simulink model "otomobil"  (Simulink 7.6)
settings: Solver=ode45  StartTime=0.0  StopTime=50  RelTol=1e-3
values from neighbouring files (symbols this model uses):
  co1 = 2500    [car.m]    (also in car_sis.m)
  co3 = 2500    [car.m]    (also in car_sis.m)
  co5 = 2500    [car.m]    (also in car_sis.m)
  co7 = 2500    [car.m]    (also in car_sis.m)
  dy = 0.007    [car.m]
  ko1 = 15000    [car.m]    (also in car_sis.m)
  ko2 = 250000    [car.m]    (also in car_sis.m)
  ko3 = 17000    [car.m]    (also in car_sis.m)
  ko4 = 250000    [car.m]    (also in car_sis.m)
  ko5 = 15000    [car.m]    (also in car_sis.m)
  ko6 = 250000    [car.m]    (also in car_sis.m)
  ko7 = 17000    [car.m]    (also in car_sis.m)
  ko8 = 250000    [car.m]    (also in car_sis.m)
  lo1 = 1.2    [car.m]
  lo2 = 1.4    [car.m]
  lo3 = 0.5    [car.m]
  lo4 = 1    [car.m]
  mo1 = 1100+80*4    (= 1420)    [car.m]    (also in car_sis.m = 1100)
  mo2 = 25    [car.m]    (also in car_sis.m)
  mo3 = 25    [car.m]    (also in car_sis.m = 45)
  mo4 = 45    [car.m]    (also in car_sis.m = 25)
  mo5 = 45    [car.m]    (also in car_sis.m)
  Vo = 50    [car.m]    (also in car_sis.m = 16.6666666667)
  wo = Vo/dy    (= 7142.85714286)    [car.m]
settings Model: Creator=user  LastModifiedBy=user

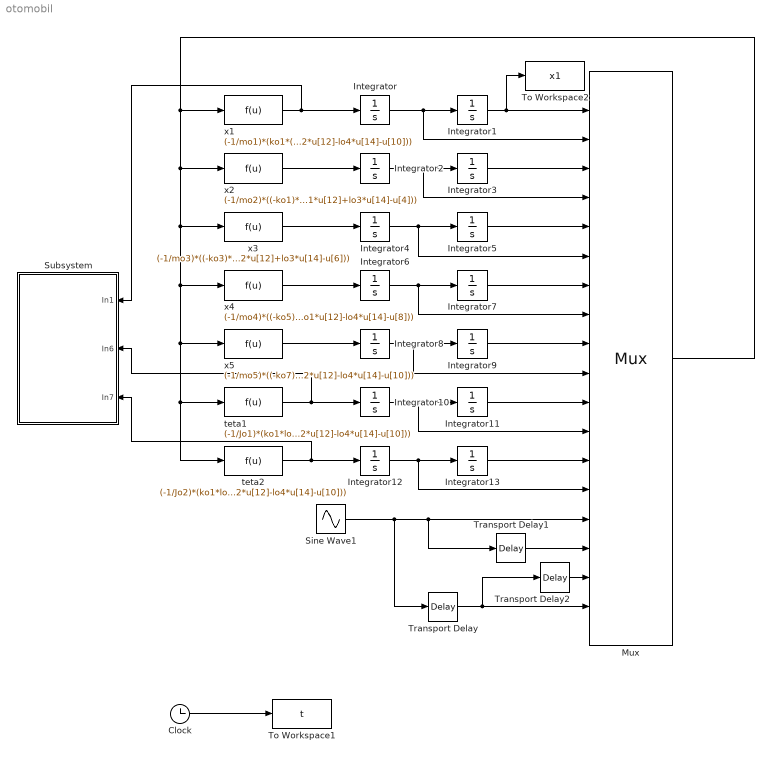
== system otomobil ==
  Clock : Clock
      settings: Decimation=10
  Integrator{,1..13} (14 alike) : Integrator
  Mux : Mux  Inputs=18
  Sine Wave1 : Sin  Amplitude=dy  Frequency=wo*2*pi  SampleTime=0
  Subsystem : Subsystem
  To Workspace1 : ToWorkspace  VariableName=t  SampleTime=-1  SaveFormat=Array
  To Workspace2 : ToWorkspace  VariableName=x1  SampleTime=-1  SaveFormat=Array
  Transport Delay : TransportDelay  DelayTime=(lo1+lo2)/Vo
  Transport Delay1 : TransportDelay  DelayTime=0.001
  Transport Delay2 : TransportDelay  DelayTime=0.001
  teta1 : Fcn  Expr=(-1/Jo1)*(ko1*lo1*(u[1]+lo1*u[11]+lo3*u[13]-u[3])-ko3*lo2*(u[1]-lo2*u[11]+lo3*u[13]-u[5])+ko5*lo1*(u[1]+lo1*u[11]-lo4*u[13]-u[7])-ko7*lo2*(u[1]-lo2*u[11]-lo4*u[13]-u[9])+co1*lo1*(u[2]+lo1*u[12]+lo3*u[14]-u[4])-co3*lo2*(u[2]-lo2*u[12]+lo3*u[14]-u[6])+co5*lo1*(u[2]+lo1*u[12]-lo4*u[14]-u[8])-co7*lo2*(u[2]-lo2*u[12]-lo4*u[14]-u[10]))
  teta2 : Fcn  Expr=(-1/Jo2)*(ko1*lo3*(u[1]+lo1*u[11]+lo3*u[13]-u[3])+ko3*lo3*(u[1]-lo2*u[11]+lo3*u[13]-u[5])-ko5*lo4*(u[1]+lo1*u[11]-lo4*u[13]-u[7])-ko7*lo4*(u[1]-lo2*u[11]-lo4*u[13]-u[9])+co1*lo3*(u[2]+lo1*u[12]+lo3*u[14]-u[4])+co3*lo3*(u[2]-lo2*u[12]+lo3*u[14]-u[6])-co5*lo4*(u[2]+lo1*u[12]-lo4*u[14]-u[8])-co7*lo4*(u[2]-lo2*u[12]-lo4*u[14]-u[10]))
  x1 : Fcn  Expr=(-1/mo1)*(ko1*(u[1]+lo1*u[11]+lo3*u[13]-u[3])+ko3*(u[1]-lo2*u[11]+lo3*u[13]-u[5])+ko5*(u[1]+lo1*u[11]-lo4*u[13]-u[7])+ko7*(u[1]-lo2*u[11]-lo4*u[13]-u[9])+co1*(u[2]+lo1*u[12]+lo3*u[14]-u[4])+co3*(u[2]-lo2*u[12]+lo3*u[14]-u[6])+co5*(u[2]+lo1*u[12]-lo4*u[14]-u[8])+co7*(u[2]-lo2*u[12]-lo4*u[14]-u[10]))
  x2 : Fcn  Expr=(-1/mo2)*((-ko1)*(u[1]+lo1*u[11]+lo3*u[13]-u[3])+ko2*(u[3]-u[15])-co1*(u[2]+lo1*u[12]+lo3*u[14]-u[4]))
  x3 : Fcn  Expr=(-1/mo3)*((-ko3)*(u[1]-lo2*u[11]+lo3*u[13]-u[5])+ko4*(u[5]-u[16])-co3*(u[2]-lo2*u[12]+lo3*u[14]-u[6]))
  x4 : Fcn  Expr=(-1/mo4)*((-ko5)*(u[1]+lo1*u[11]-lo4*u[13]-u[7])+ko6*(u[7]-u[17])-co5*(u[2]+lo1*u[12]-lo4*u[14]-u[8]))
  x5 : Fcn  Expr=(-1/mo5)*((-ko7)*(u[1]-lo2*u[11]-lo4*u[13]-u[9])+ko8*(u[5]-u[18])-co7*(u[2]-lo2*u[12]-lo4*u[14]-u[10]))
  wires:
  x1/1 -> Integrator/1, Subsystem/1(In1)
  Integrator/1 -> Integrator1/1, Mux/2
  x2/1 -> Integrator2/1
  Integrator2/1 -> Integrator3/1, Mux/4
  x3/1 -> Integrator4/1
  Integrator4/1 -> Integrator5/1, Mux/6
  x4/1 -> Integrator6/1
  Integrator6/1 -> Integrator7/1, Mux/8
  x5/1 -> Integrator8/1
  Integrator8/1 -> Integrator9/1, Mux/10
  teta1/1 -> Integrator10/1, Subsystem/2(In6)
  Integrator10/1 -> Integrator11/1, Mux/12
  teta2/1 -> Integrator12/1, Subsystem/3(In7)
  Integrator12/1 -> Integrator13/1, Mux/14
  Integrator3/1 -> Mux/3
  Integrator5/1 -> Mux/5
  Integrator7/1 -> Mux/7
  Integrator9/1 -> Mux/9
  Integrator11/1 -> Mux/11
  Integrator13/1 -> Mux/13
  Integrator1/1 -> Mux/1, To Workspace2/1
  Mux/1 -> x1/1, x2/1, x4/1, x5/1, teta2/1, teta1/1, x3/1
  Sine Wave1/1 -> Mux/15, Transport Delay1/1, Transport Delay/1
  Transport Delay/1 -> Mux/18, Transport Delay2/1
  Clock/1 -> To Workspace1/1
  Transport Delay1/1 -> Mux/16
  Transport Delay2/1 -> Mux/17

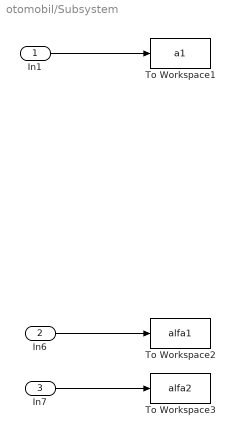
== system otomobil/Subsystem ==
  In1 : Inport
  In6 : Inport  Port=2
  In7 : Inport  Port=3
  To Workspace1 : ToWorkspace  VariableName=a1  SampleTime=-1  SaveFormat=Array
  To Workspace2 : ToWorkspace  VariableName=alfa1  SampleTime=-1  SaveFormat=Array
  To Workspace3 : ToWorkspace  VariableName=alfa2  SampleTime=-1  SaveFormat=Array
  wires:
  In1/1 -> To Workspace1/1
  In6/1 -> To Workspace2/1
  In7/1 -> To Workspace3/1
